simulink model "Software_Sensing"  (R2020a)
settings: Solver=FixedStepAuto  StartTime=0.0  StopTime=1  FixedStep=1e-3  RelTol=1e-3  EnableMultiTasking=on
model workspace (MAT data in the model file):
  duty_cycle = 5
settings Model: ExtModeTrigDuration=5  Creator=theodor  LastModifiedBy=theodor
settings OptimizationCC: EnhancedBackFolding=on  PassReuseOutputArgsAs=Individual arguments  ZeroExternalMemoryAtStartup=off  ZeroInternalMemoryAtStartup=off  MaxStackSize=64  OptimizeBlockOrder=speed  DifferentSizesBufferReuse=on  OptimizationCustomize=off  EfficientTunableParamExpr=on
settings DebuggingCC: ParameterTunabilityLossMsg=error
settings HardwareCC: ProdBitPerPointer=32  ProdBitPerSizeT=32  ProdBitPerPtrDiffT=32  ProdLargestAtomicInteger=Long  ProdLargestAtomicFloat=Double  ProdWordSize=32  ProdHWDeviceType=ARM Compatible->ARM Cortex
settings SFSimCC: MATLABDynamicMemAlloc=off
settings RTWCC: SystemTargetFile=ert.tlc  HardwareBoard=NXP FRDM-K64F  TemplateMakefile=ert_default_tmf  Toolchain=GNU Tools for ARM Embedded Processors
settings CodeAppCC: ForceParamTrailComments=on  IgnoreCustomStorageClasses=off  OperatorAnnotations=on  SimulinkDataObjDesc=on  SFDataObjDesc=on  InsertBlockDesc=on

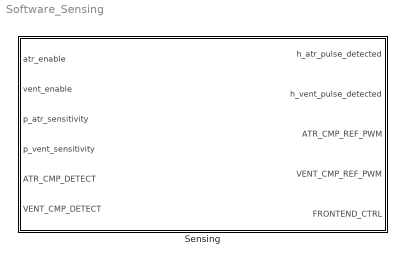
== system Software_Sensing ==
  Sensing : Subsystem

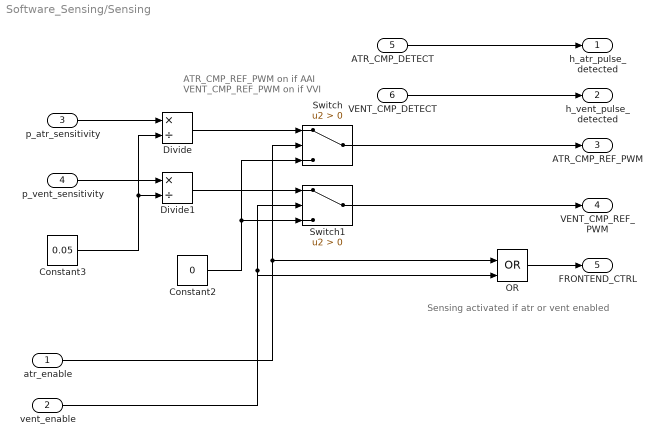
== system Software_Sensing/Sensing ==
  note: ATR_CMP_REF_PWM on if AAI
      | VENT_CMP_REF_PWM on if VVI
  note: Sensing activated if atr or vent enabled
  atr_enable : Inport
  vent_enable : Inport  Port=2
  p_atr_sensitivity : Inport  Port=3
  p_vent_sensitivity : Inport  Port=4
  ATR_CMP_DETECT : Inport  Port=5
  VENT_CMP_DETECT : Inport  Port=6
  Constant2 : Constant  Value=0
  Constant3 : Constant  Value=0.05
  Divide : Product  Inputs=*/
  Divide1 : Product  Inputs=*/
  OR : Logic  Operator=OR  IconShape=distinctive  AllPortsSameDT=off  OutDataTypeStr=boolean
  Switch : Switch  Criteria=u2 > Threshold
  Switch1 : Switch  Criteria=u2 > Threshold
  h_atr_pulse_detected : Outport
  h_vent_pulse_detected : Outport  Port=2
  ATR_CMP_REF_PWM : Outport  Port=3
  VENT_CMP_REF_PWM : Outport  Port=4
  FRONTEND_CTRL : Outport  Port=5
  wires:
  OR/1 -> FRONTEND_CTRL/1
  atr_enable/1 -> OR/1, Switch/2
  Switch/1 -> ATR_CMP_REF_PWM/1
  Switch1/1 -> VENT_CMP_REF_PWM/1
  ATR_CMP_DETECT/1 -> h_atr_pulse_detected/1
  VENT_CMP_DETECT/1 -> h_vent_pulse_detected/1
  Constant2/1 -> Switch/3, Switch1/3
  p_atr_sensitivity/1 -> Divide/1
  Divide/1 -> Switch/1
  Divide1/1 -> Switch1/1
  p_vent_sensitivity/1 -> Divide1/1
  Constant3/1 -> Divide1/2, Divide/2
  vent_enable/1 -> OR/2, Switch1/2
